simulink model "s0435"  (Simulink 7.0)
settings: Solver=ode3  SolverMode=SingleTasking  StartTime=0.0  StopTime=900  FixedStep=1  MaxStep=1  RelTol=1e-3  AbsTol=1e-6
values from neighbouring files (symbols this model uses):
  Kpr = 10    [m0108d.m]    (also in m0109b.m = 1; m0113c.m; m0404Bsp.m = 3)
  t0A = -1    [m0404Bsp.m]
undefined symbols (not defined in the file or in its folder): eab, ean, edach, Tr
settings Model: Creator=froriep  LastModifiedBy=froriep
settings DataIOCC: LimitDataPoints=off  SaveOutput=off  SaveTime=off
settings OptimizationCC: BooleanDataType=off
settings DebuggingCC: SaveWithParameterizedLinksMsg=none  SignalResolutionControl=TryResolveAllWithWarning  SolverPrmCheckMsg=none  MultiTaskDSMMsg=warning  MultiTaskCondExecSysMsg=none  StrictBusMsg=None
settings HardwareCC: TargetUnknown=on
settings RTWCC: IncludeERTFirstTime=on

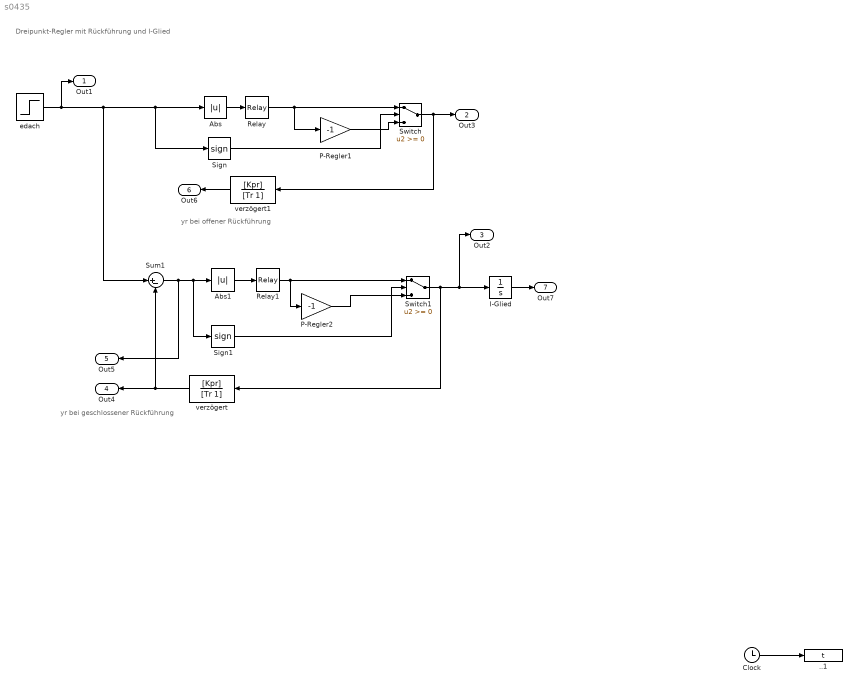
== system s0435 ==
  note: Dreipunkt-Regler mit Rückführung und I-Glied
  note: yr bei offener Rückführung
  note: yr bei geschlossener Rückführung
  ..1 : ToWorkspace  VariableName=t  SaveFormat=Array
  Abs : Abs  OutDataType=sfix(16)  OutScaling=2^0
  Abs1 : Abs  OutDataType=sfix(16)  OutScaling=2^0
  Clock : Clock
      settings: Decimation=10
  I-Glied : Integrator
  P-Regler1 : Gain  Gain=-1  ParameterDataType=sfix(16)  ParameterScaling=2^0  OutDataType=sfix(16)  OutScaling=2^0
  P-Regler2 : Gain  Gain=-1  ParameterDataType=sfix(16)  ParameterScaling=2^0  OutDataType=sfix(16)  OutScaling=2^0
  Relay : Relay  OnSwitchValue=ean  OffSwitchValue=eab  OnOutputValue=Yh  OutDataType=sfix(16)  OutScaling=2^0
  Relay1 : Relay  OnSwitchValue=ean  OffSwitchValue=eab  OnOutputValue=Yh  OutDataType=sfix(16)  OutScaling=2^0
  Sign : Signum
  Sign1 : Signum
  Sum1 : Sum  Inputs=|+-  SaturateOnIntegerOverflow=on  InputSameDT=on
  Switch : Switch  OutDataType=sfix(16)  OutScaling=2^0
  Switch1 : Switch  OutDataType=sfix(16)  OutScaling=2^0
  edach : Step  Time=-t0A  After=edach  SampleTime=0
  verzögert : TransferFcn  Orientation=left  Numerator=[Kpr]  Denominator=[Tr 1]
  verzögert1 : TransferFcn  Orientation=left  Numerator=[Kpr]  Denominator=[Tr 1]
  Out1 : Outport  OutDataType=sfix(16)  OutScaling=2^0
  Out3 : Outport  Port=2  OutDataType=sfix(16)  OutScaling=2^0
  Out2 : Outport  Port=3  OutDataType=sfix(16)  OutScaling=2^0
  Out4 : Outport  Orientation=left  Port=4  OutDataType=sfix(16)  OutScaling=2^0
  Out5 : Outport  Orientation=left  Port=5  OutDataType=sfix(16)  OutScaling=2^0
  Out6 : Outport  Orientation=left  Port=6  OutDataType=sfix(16)  OutScaling=2^0
  Out7 : Outport  Port=7  OutDataType=sfix(16)  OutScaling=2^0
  wires:
  Clock/1 -> ..1/1
  Sum1/1 -> Out5/1, Abs1/1, Sign1/1
  verzögert/1 -> Sum1/2, Out4/1
  Switch/1 -> Out3/1, verzögert1/1
  Abs/1 -> Relay/1
  Sign/1 -> Switch/2
  Relay/1 -> Switch/1, P-Regler1/1
  P-Regler1/1 -> Switch/3
  Abs1/1 -> Relay1/1
  Switch1/1 -> verzögert/1, Out2/1, I-Glied/1
  verzögert1/1 -> Out6/1
  Relay1/1 -> Switch1/1, P-Regler2/1
  P-Regler2/1 -> Switch1/3
  Sign1/1 -> Switch1/2
  edach/1 -> Abs/1, Sign/1, Sum1/1, Out1/1
  I-Glied/1 -> Out7/1
